simulink model "test"  (R2020a)
settings: Solver=VariableStepAuto  StartTime=0.0  StopTime=10.0  RelTol=1e-3
libraries: sharedtransform x3, aerolibutil x1
settings Model: Creator=thomas  LastModifiedBy=thomas

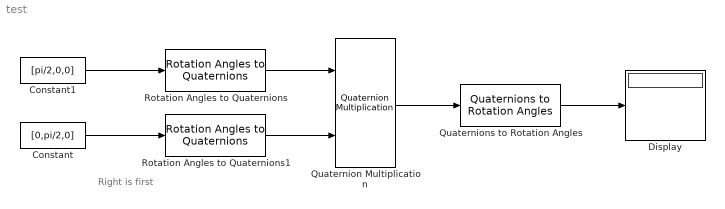
== system test ==
  note: Right is first
  Constant : Constant  Value=[0,pi/2,0]
  Constant1 : Constant  Value=[pi/2,0,0]
  Display : Display
  Quaternion Multiplication : aerolibutil/Quaternion Multiplication
  Quaternions to Rotation Angles : sharedtransform/Quaternions to Rotation Angles  rotationOrder=YZX  aMode=aMode
      settings: SourceProductBaseCode=AE,PW,MT,VE,VP
  Rotation Angles to Quaternions : sharedtransform/Rotation Angles to Quaternions  rotationOrder=YZX  aMode=aMode
      settings: SourceProductBaseCode=AE,PW,MT,VE,VP
  Rotation Angles to Quaternions1 : sharedtransform/Rotation Angles to Quaternions  rotationOrder=YZX  aMode=aMode
      settings: SourceProductBaseCode=AE,PW,MT,VE,VP
  wires:
  Rotation Angles to Quaternions/1 -> Quaternion Multiplication/1
  Rotation Angles to Quaternions1/1 -> Quaternion Multiplication/2
  Quaternion Multiplication/1 -> Quaternions to Rotation Angles/1
  Quaternions to Rotation Angles/1 -> Display/1
  Constant/1 -> Rotation Angles to Quaternions1/1
  Constant1/1 -> Rotation Angles to Quaternions/1
